simulink library "tru"  (Simulink 8.1)
settings: Solver=ode1  StartTime=0.0  StopTime=Inf  FixedStep=0.001  RelTol=1e-3
PostLoadFcn:
  | , if any(exist('dsrtsu_mdlpostloadfcn', 'file') == [2, 3, 6]), try dsrtsu_mdlpostloadfcn('Execute', bdroot); catch fprintf('Error in PostLoadFcn (dsrtsu_mdlpostloadfcn) for model "%s":\n %s\n', bdroot, lasterr); end, end,
undefined symbols (not defined in the file or in its folder): C_TICK_TIME_S, KACC_ACCTorqueIncSteps_num, KACC_ACCTorqueIncTimer_s, TRUE, ZERO_INT
settings Model: DSRTSU_INTERNAL_RTI_VER=450  DSRTSU_INTERNAL_RTI_TYPE=rti1401  RTICANMMDATA=struct('GeneralSetupData',struct('modelroot','D:\ELN150201_TAIWAN\trunk\AdasDragon\software\sw_development\arch\app\acc','generalsettings',struct('filesettings',struct('destfolder',struct('Name','RTICANMM_FILES','Check',1),'buildfolder',struct('Name','.','Check',1),'AbsDestfolder',struct('Name','D:\ELN150201_TAIWAN\trunk\AdasDragon\software\sw_development\arch\app\acc\RTICANMM_FILES'),'AbsBuildfolder',struct('Name','D:\ELN150201_TAIWAN\trunk\AdasDragon\software\sw_development\arch\app\acc'))),'options',struct('addpaths',1,'rmpaths',1,'addtrcexclusion',logical(1),'cannavigator',struct('checkmonitoring',0),'show_usrtrc',0,'use_usrtrc',0),'advanced',struct('options',[1 1 1 1 1 1 1 1 1 1 1 1 1 1 1 1 1 1 1 1 1 1 1 1 1 1 1 1 1 1 1 1 1 1 1 1 1 1 1 1 1 1 1 1 1 1 1 1 1 1 1 1 1 1 1 1 1 1 1 1 1 1 1 1 1 1 1 1 1 1 1 1 1 1 1 1 1 1 1 1 1 1 1 1 1 1 1 1 1 1 1 1 1 1 1 1 1 1 1 1]),'MPSetup',{{}},'modelname','tru','block','tru'))  DSRTSU_INTERNAL_RTIFPGA=40  Creator=AT015555  LastModifiedBy=AT015555

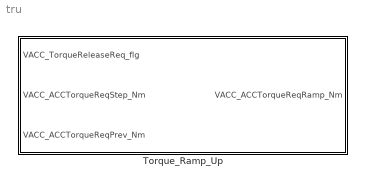
== system tru ==
  Torque_Ramp_Up : Subsystem

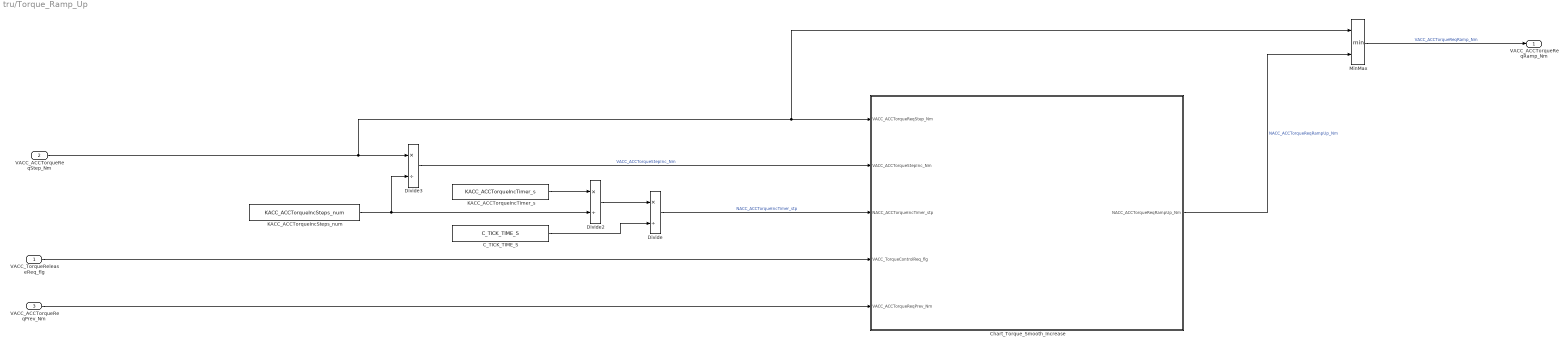
== system tru/Torque_Ramp_Up ==
  VACC_TorqueReleaseReq_flg : Inport
  VACC_ACCTorqueReqStep_Nm : Inport  Port=2
  VACC_ACCTorqueReqPrev_Nm : Inport  Port=3
  C_TICK_TIME_S : Constant  Value=C_TICK_TIME_S
  Chart_Torque_Smooth_Increase : Stateflow chart  TreatAsAtomicUnit=on
  Divide : Product  Inputs=*/
  Divide2 : Product  Inputs=*/
  Divide3 : Product  Inputs=*/
  KACC_ACCTorqueIncSteps_num : Constant  Value=KACC_ACCTorqueIncSteps_num
  KACC_ACCTorqueIncTimer_s : Constant  Value=KACC_ACCTorqueIncTimer_s
  MinMax : MinMax  Inputs=2
  VACC_ACCTorqueReqRamp_Nm : Outport
  wires:
  VACC_ACCTorqueReqPrev_Nm/1 -> Chart_Torque_Smooth_Increase/5(VACC_ACCTorqueReqPrev_Nm)
  Chart_Torque_Smooth_Increase/1(NACC_ACCTorqueReqRampUp_Nm) -> MinMax/2  "NACC_ACCTorqueReqRampUp_Nm"
  Divide3/1 -> Chart_Torque_Smooth_Increase/2(VACC_ACCTorqueStepInc_Nm)  "VACC_ACCTorqueStepInc_Nm"
  KACC_ACCTorqueIncSteps_num/1 -> Divide2/2, Divide3/2
  KACC_ACCTorqueIncTimer_s/1 -> Divide2/1
  Divide/1 -> Chart_Torque_Smooth_Increase/3(NACC_ACCTorqueIncTimer_stp)  "NACC_ACCTorqueIncTimer_stp"
  C_TICK_TIME_S/1 -> Divide/2
  Divide2/1 -> Divide/1
  VACC_ACCTorqueReqStep_Nm/1 -> Chart_Torque_Smooth_Increase/1(VACC_ACCTorqueReqStep_Nm), MinMax/1, Divide3/1
  MinMax/1 -> VACC_ACCTorqueReqRamp_Nm/1  "VACC_ACCTorqueReqRamp_Nm"
  VACC_TorqueReleaseReq_flg/1 -> Chart_Torque_Smooth_Increase/4(VACC_TorqueControlReq_flg)

== stateflow chart Torque_Ramp_Up/Chart_Torque_Smooth_Increase ==
  state INIT_TQ
    en:
    NACC_ACCTorqueReqRampUp_Nm = VACC_ACCTorqueReqPrev_Nm;
  state COUNT
    en:
    NACC_ACCTorqueIncTimerLocal_stp=ZERO_INT;
    du:
    NACC_ACCTorqueIncTimerLocal_stp=NACC_ACCTorqueIncTimerLocal_stp+1;
  state INC_TQ
    en:
    NACC_ACCTorqueReqRampUp_Nm=NACC_ACCTorqueReqRampUp_Nm+VACC_ACCTorqueStepInc_Nm;
  (default) -> INIT_TQ
  COUNT -> INC_TQ [order 1] : [NACC_ACCTorqueIncTimerLocal_stp>NACC_ACCTorqueIncTimer_stp...
      | && NACC_ACCTorqueReqRampUp_Nm<VACC_ACCTorqueReqStep_Nm]
  INIT_TQ -> COUNT : [NACC_ACCTorqueReqRampUp_Nm<VACC_ACCTorqueReqStep_Nm]
  INC_TQ -> COUNT [order 1] : [NACC_ACCTorqueReqRampUp_Nm<VACC_ACCTorqueReqStep_Nm]
  COUNT -> INIT_TQ [order 2] : [VACC_TorqueControlReq_flg==TRUE]
  INC_TQ -> INIT_TQ [order 2] : [VACC_TorqueControlReq_flg==TRUE]
  data: VACC_ACCTorqueReqStep_Nm input double; VACC_ACCTorqueStepInc_Nm input double; NACC_ACCTorqueIncTimer_stp input double; NACC_ACCTorqueReqRampUp_Nm output single; NACC_ACCTorqueIncTimerLocal_stp local single; ZERO_INT parameter uint8; VACC_TorqueControlReq_flg input double; TRUE parameter boolean; VACC_ACCTorqueReqPrev_Nm input double
